simulink model "control"  (R2022b)
settings: Solver=VariableStepAuto  StartTime=0.0  StopTime=4  RelTol=1e-3
undefined symbols (not defined in the file or in its folder): DiscIntNeverNeededParam
libraries: matrix_library x2
settings Model: Creator=giuseppeloianno  LastModifiedBy=reube
settings DataIOCC: ReturnWorkspaceOutputs=off

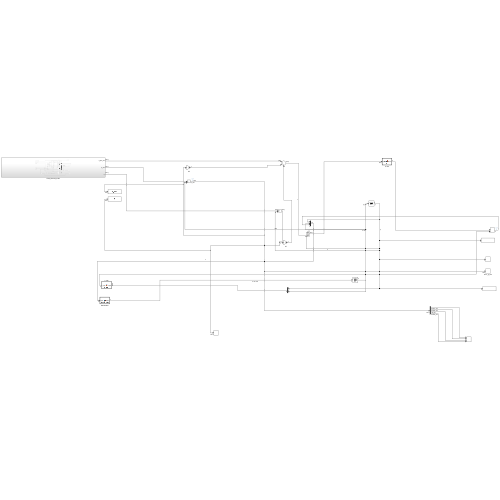
[thumbnail: Simulink's stored preview of the top-level diagram]
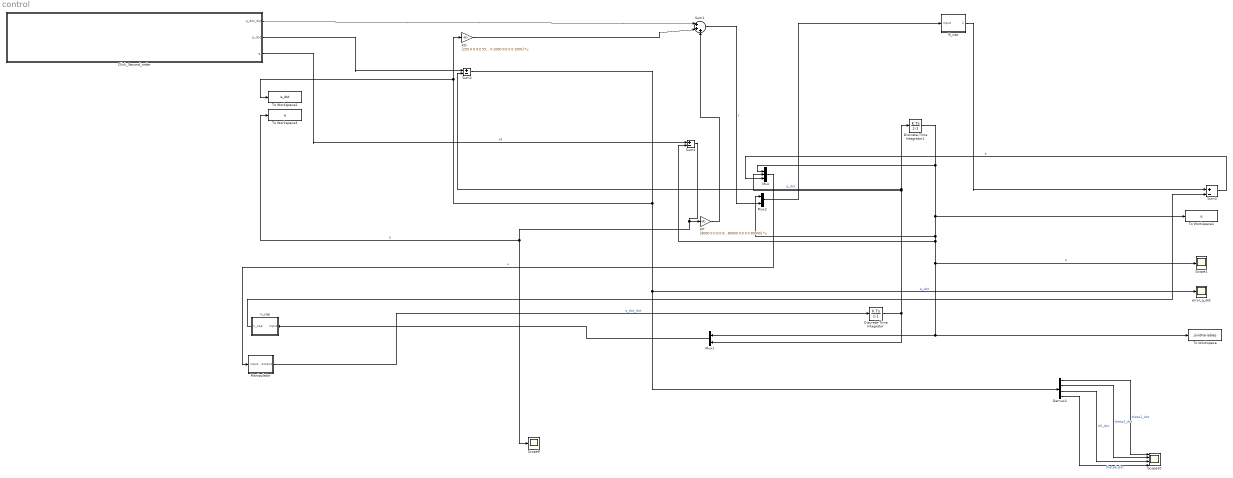
== system control ==
  B_cap : MATLAB Function  TreatAsAtomicUnit=on
  Click_Second_order : Subsystem
  Demux2 : Demux
  Discrete-Time Integrator : DiscreteIntegrator  InitialCondition=[0;0;0;0]  SampleTime=0.001  ICPrevOutput=DiscIntNeverNeededParam  ICPrevScaledInput=DiscIntNeverNeededParam
  Discrete-Time Integrator1 : DiscreteIntegrator  InitialCondition=[-0.9273;-1.2870;0.700;2.2143]  SampleTime=0.001  ICPrevOutput=DiscIntNeverNeededParam  ICPrevScaledInput=DiscIntNeverNeededParam
  KD : Gain  Gain=[250 0 0 0;0 550 0 0;0 0 1000 0;0 0 0 1000]  Multiplication=Matrix(K*u) (u vector)
  KP : Gain  Gain=[8000 0 0 0;0 8000 0 0;0 0 80000 0;0 0 0 80000]  Multiplication=Matrix(K*u) (u vector)
  Manipulator : MATLAB Function  TreatAsAtomicUnit=on
  Mux : Mux  Inputs=3
  Mux1 : Mux  Inputs=2
  Mux2 : Mux  Inputs=2
  Scope1 : Scope
  Scope10 : Scope  NumInputPorts=4
  Scope9 : Scope
  Sum1 : Sum  Inputs=|+++
  Sum2 : Sum  Inputs=|+-
  Sum3 : Sum  Inputs=|+-
  Sum4 : Sum  Inputs=|+-
  To Workspace : ToWorkspace  VariableName=jointVariables  SampleTime=-1
  To Workspace1 : ToWorkspace  VariableName=q  SampleTime=-1
  To Workspace2 : ToWorkspace  VariableName=e_dot  SampleTime=-1
  To Workspace3 : ToWorkspace  VariableName=e  SampleTime=-1
  error_q_dot : Scope
  n_cap : MATLAB Function  TreatAsAtomicUnit=on
  wires:
  Mux/1 -> Manipulator/1(input)  "u"
  Demux2/1 -> Scope10/1  "theta1_dot"
  n_cap/1(n_cap) -> Sum3/2
  Sum1/1 -> Mux2/2  "y"
  B_cap/1(Bmatrixtrue) -> Sum3/1
  Demux2/2 -> Scope10/2  "theta2_dot"
  Sum2/1 -> Demux2/1, error_q_dot/1, To Workspace2/1, KD/1  "e_dot"
  Discrete-Time Integrator1/1 -> Mux1/1, To Workspace/1, Scope1/1, Sum4/2, Mux2/1, To Workspace1/1, Mux/1  "q"
  Mux1/1 -> n_cap/1(input)
  Demux2/3 -> Scope10/3  "d3_dot"
  Manipulator/1(output) -> Discrete-Time Integrator/1  "q_dot_dot"
  Discrete-Time Integrator/1 -> Sum2/2, Discrete-Time Integrator1/1, Mux/2, Mux1/2  "q_dot"
  KD/1 -> Sum1/2
  Click_Second_order/3(q) -> Sum4/1  "xd"
  Sum3/1 -> Mux/3  "e"
  Click_Second_order/2(q_dot) -> Sum2/1
  Sum4/1 -> To Workspace3/1, Scope9/1, KP/1  "e"
  Mux2/1 -> B_cap/1(input)
  Demux2/4 -> Scope10/4  "theta4_dot"
  Click_Second_order/1(q_dot_dot) -> Sum1/1
  KP/1 -> Sum1/3

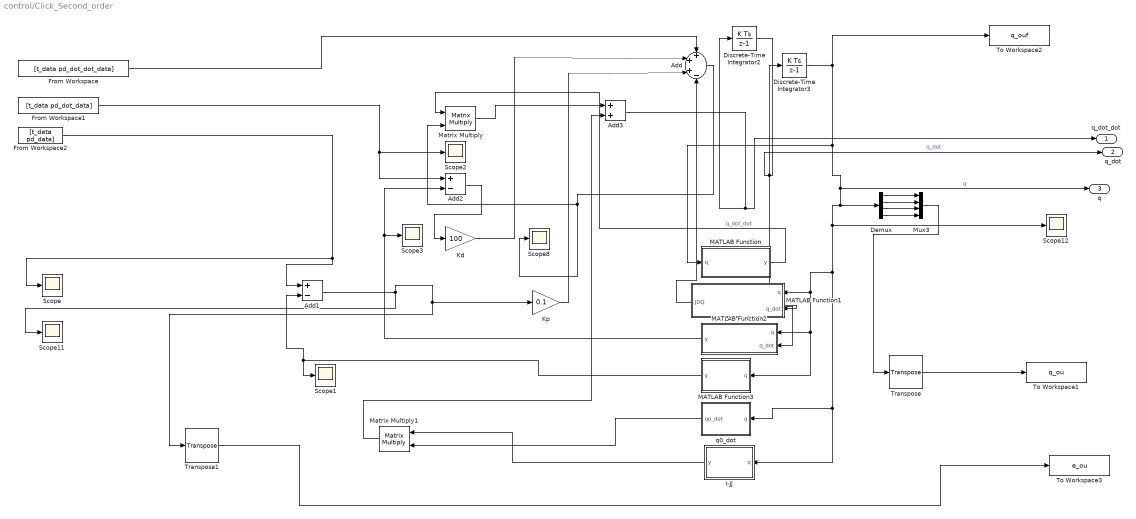
== system control/Click_Second_order ==
  Add : Sum  Inputs=+++-
  Add1 : Sum  Inputs=+-
  Add2 : Sum  Inputs=+-
  Add3 : Sum
  Demux : Demux
  Discrete-Time Integrator2 : DiscreteIntegrator  InitialCondition=[-0.927293431584587;-1.287005790420619;0.700000000000000;2.214299222005206]  SampleTime=0.001  LimitOutput=on  UpperSaturationLimit=[pi/2 pi/4 1 2*pi]'  LowerSaturationLimit="[-pi/2 -pi/2 0.25  -2*pi]'"  ICPrevOutput=DiscIntNeverNeededParam  ICPrevScaledInput=DiscIntNeverNeededParam
  Discrete-Time Integrator3 : DiscreteIntegrator  InitialCondition=[-0.9273;-1.2870;0.700;2.2143]  SampleTime=0.001  LimitOutput=on  UpperSaturationLimit=[pi/2 pi/4 1 2*pi]'  LowerSaturationLimit="[-pi/2 -pi/2 0.25  -2*pi]'"  ICPrevOutput=DiscIntNeverNeededParam  ICPrevScaledInput=DiscIntNeverNeededParam
  From Workspace : FromWorkspace  VariableName=[t_data pd_dot_dot_data]  SampleTime=0.001
  From Workspace1 : FromWorkspace  VariableName=[t_data pd_dot_data]  SampleTime=0.001
  From Workspace2 : FromWorkspace  VariableName=[t_data pd_data]  SampleTime=0.001
  I-JJ : MATLAB Function  TreatAsAtomicUnit=on
  Kd : Gain  Gain=100
  Kp : Gain  Gain=0.1
  MATLAB Function : MATLAB Function  TreatAsAtomicUnit=on
  MATLAB Function1 : MATLAB Function  TreatAsAtomicUnit=on
  MATLAB Function2 : MATLAB Function  TreatAsAtomicUnit=on
  MATLAB Function3 : MATLAB Function  TreatAsAtomicUnit=on
  Matrix Multiply : Product  Multiplication=Matrix(*)
  Matrix Multiply1 : Product  Multiplication=Matrix(*)
  Mux3 : Mux
  Scope{,1..3,8,11..12} (7 alike) : Scope
  To Workspace1 : ToWorkspace  VariableName=q_ou  SampleTime=-1
      settings: Save2DSignal=2-D array (concatenate along first dimension)
  To Workspace2 : ToWorkspace  VariableName=q_ouf  SampleTime=-1
  To Workspace3 : ToWorkspace  VariableName=e_ou  SampleTime=-1
      settings: Save2DSignal=2-D array (concatenate along first dimension)
  Transpose : matrix_library/Transpose
  Transpose1 : matrix_library/Transpose
  q0_dot : MATLAB Function  TreatAsAtomicUnit=on
  q_dot_dot : Outport
  q_dot : Outport  Port=2
  q : Outport  Port=3
  wires:
  Demux/1 -> Mux3/1
  From Workspace/1 -> Add/1
  Demux/2 -> Mux3/2
  Matrix Multiply1/1 -> Add3/2
  Discrete-Time Integrator2/1 -> q_dot/1, MATLAB Function2/2(q_dot), MATLAB Function1/2(q_dot), Discrete-Time Integrator3/1  "q_dot"
  I-JJ/1(y) -> Matrix Multiply1/1
  MATLAB Function1/1(JDQ) -> Add/4
  Add2/1 -> Kd/1
  Kd/1 -> Add/2
  Demux/3 -> Mux3/3
  Matrix Multiply/1 -> Add3/1
  Discrete-Time Integrator3/1 -> q/1, Demux/1, I-JJ/1(q), q0_dot/1(q), MATLAB Function3/1(q), MATLAB Function2/1(q), MATLAB Function1/1(q), Scope12/1, MATLAB Function/1(q), To Workspace2/1  "q"
  Add1/1 -> Transpose1/1, Kp/1, Scope11/1
  MATLAB Function/1(y) -> Matrix Multiply/1  "q_dot_dot"
  MATLAB Function2/1(y) -> Add2/2, Scope3/1
  From Workspace1/1 -> Add2/1, Scope2/1
  From Workspace2/1 -> Add1/1, Scope/1
  Add/1 -> Scope8/1, Matrix Multiply/2
  Kp/1 -> Add/3
  Add3/1 -> Discrete-Time Integrator2/1, q_dot_dot/1
  MATLAB Function3/1(y) -> Add1/2, Scope1/1
  Mux3/1 -> Transpose/1
  Transpose1/1 -> To Workspace3/1
  Transpose/1 -> To Workspace1/1
  Demux/4 -> Mux3/4
  q0_dot/1(qo_dot) -> Matrix Multiply1/2

== matlab function control/Click_Second_order/MATLAB Function ==
  data: q input; y output
function y =pinvj(q)

avariable1 = 0.5;
avariable2 = 0.5;
theta1 = q(1);
theta2 = q(2);
d3 = q(3);
bsum = theta1+theta2;
c1 = cos(theta1);
s1 = sin(theta1);
c12 = cos(bsum);
s12 = sin(bsum);

J = [-avariable2*s12-avariable1*s1 -avariable2*s12 0 0; 
    avariable2*c12+avariable1*c1 avariable2*c12 0 0;  
    0 0 1 0];
x= pinv(J);
y=x;
end

== matlab function control/Click_Second_order/MATLAB Function2 ==
  data: q input; q_dot input; y output
function y = jacobian(q, q_dot)
a1 = 0.5;
a2 = 0.5;
t1 = q(1);
t2 = q(2);
d3 = q(3);
b = t1+t2;
c1 = cos(t1);
s1 = sin(t1);
c12 = cos(b);
s12 = sin(b);


J = [-a2*s12-a1*s1 -a2*s12 0 0; 
    a2*c12+a1*c1 a2*c12 0 0;  
    0 0 -1.5+d3 0];
y = J*q_dot;

end

== matlab function control/Click_Second_order/MATLAB Function3 ==
  data: q input; y output
function y = direct_kin(q)
aSIDE1=0.5;
aSIDE2=0.5;
tETA1=q(1);
tETA2=q(2);
b=tETA1+tETA2;
d3side=q(3);
ct1= cos(tETA1);
st1 = sin(tETA1);
ct12 = cos(b);
st12 = sin(b);
y=[aSIDE2*ct12+aSIDE1*ct1;
   aSIDE1*st12 + aSIDE1*st1;
   -1.5+d3side];
end

== matlab function control/Click_Second_order/I-JJ ==
  data: q input; y output
function y = ijj(q)


aside1 = 0.5;
aside2 = 0.5;
theta1 = q(1);
theta2 = q(2);
d3 = q(3);
bsum = theta1+theta2;
c1 = cos(theta1);
s1 = sin(theta1);
c12 = cos(bsum);
s12 = sin(bsum);
k = 10;

Jacobian = [-aside2*s12-aside1*s1 -aside2*s12 0 0; 
    aside2*c12+aside1*c1 aside2*c12 0 0;  
    0 0 1 0];
x= pinv(Jacobian);


c = [1 0 0 0; 0 1 0 0; 0 0 1 0; 0 0 0 1] - (x * Jacobian);

%p=[0.4;-0.7;0.5;1];


%q_dotmatrix=[-(2*(sin(bsum)/2 + sin(q(1))/2)*(cos(bsum)/2 + cos(q(1))/2 - p(1,:)) - 2*(cos(bsum)/2 + cos(q(1))/2)*(sin(bsum)/2 + sin(q(1))/2 + p(2,:)))/(2*((cos(bsum)/2 + cos(q(1))/2 - p(1,:))^2 + (sin(bsum)/2 + sin(q(1))/2 + p(2,:))^2 + (q(3) - p(3,:))^2)^(1/2)),  -(sin(bsum)*(cos(bsum)/2 + cos(q(1))/2 - p(1,:)) - cos(bsum)*(sin(bsum)/2 + sin(q(1))/2 + p(2,:)))/(2*((cos(bsum)/2 + cos(q(1))/2 - p(1,:))^2 + (sin(bsum)/2 + sin(q(1))/2 + p(2,:))^2 + (q(3) - p(3,:))^2)^(1/2)),  (2*q(3) - 1)/(2*((cos(bsum)/2 + cos(q(1))/2 - p(1,:))^2 + (sin(bsum)/2 + sin(q(1))/2 + p(2,:))^2 + (q(3) - p(3,:))^2)^(1/2)), 0];


%g =k* q_dotmatrix.';

y = c ;
end

== matlab function control/Click_Second_order/q0_dot ==
  data: q input; qo_dot output
function qo_dot = qodot(q)


aside1 = 0.5;
aside2 = 0.5;
theta1 = q(1);
theta2 = q(2);
t3 = q(3);
b = theta1+theta2;
cside1 = cos(theta1);
sside1 = sin(theta1);
cside12 = cos(b);
sside12 = sin(b);
k = 10;

J = [-aside2*sside12-aside1*sside1 -aside2*sside12 0 0; 
    aside2*cside12+aside1*cside1 aside2*cside12 0 0;  
    1 1 0 1];
x= pinv(J);


c = [1 0 0 0; 0 1 0 0; 0 0 1 0; 0 0 0 1] - (x * J);

p=[0.4;-0.7;0.5;1];
p1= p(1);
p2=p(2);
p3=p(3);

qo_dot=k * [(-q(1)/(4*(pi)^2));(-4/(9*(pi)^2))*(q(2)+(pi*8));(0.625-q(3))/2.25;-q(4)/(16*(pi)^2)];

end

== matlab function control/B_cap ==
  data: input input; Bmatrixtrue output
function  Bmatrixtrue = B(input)
    t2=input(2,:);
    yinput1=input(5,:);
    yinput2=input(6,:);
    yinput3=input(7,:);    
    yinput4=input(8,:);
    massl1 = 25;
    massl2 = 25;
    massl3 = 10;
    massl4 = 0;
    Ilink1 = 5;
    Ilink2 = 5;
    Ilink4 = 1;
    Imass1 = 0.0001;
    Imass2 = 0.0001;
    Imass3 = 0.01;
    Imass4 = 0.005;
    l1 = 0.25;
    l2 = 0.25;
    kinetic1 = 1;
    kinetic2 = 1;
    kinetic3 = 50;
    kinetic4 = 20;
    g = 9.8;
    b11=l1^2*massl1+(0.25+l2^2+l2*cos(t2))*massl2+(0.5+0.5*cos(t2))*(massl3+massl4)+Ilink1+Ilink2+Ilink4+Imass1*kinetic1^2+Imass2+Imass3+Imass4;
    b12=(0.5*l2*cos(t2)+l2^2)*massl2+(0.25+0.25*cos(t2))*(massl3+massl4)+Ilink2+Ilink4+Imass2*kinetic2++Imass3+Imass4;
    b13=-kinetic3*Imass3;
    b14=kinetic4*Imass4+Ilink4;
    b21=b12;
    b22=l2^2*massl2+0.25*(massl4+massl3)+Ilink2+Ilink4+Imass2*kinetic2^2+Imass4+Imass3;
    b23=-kinetic3*Imass3;
    b24=kinetic4*Imass4+Ilink4;
    b31=b13;
    b32=b23;
    b33=Imass3*kinetic3^2+massl3+massl4;
    b34=0;
    b41=b14;
    b42=b24;
    b43=b34;
    b44=Imass4*kinetic4^2+Ilink4;
    Bmatrixt=[b11 b12 b13 b14; b21 b22 b23 b24; b31 b32 b33 b34; b41 b42 b43 b44];
    Bmatrixtrue=Bmatrixt*transpose([yinput1 yinput2 yinput3 yinput4]);
end

== matlab function control/Manipulator ==
  data: input input; output output
function output = Manipulator(input)
% Part 2 manipulatort2d
   t1 = input(1,:);
    t2 = input(2,:);
    d3 = input(3,:);
    t4 = input(4,:);
    t1d = input(5,:);
    t2d = input(6,:);
    d3d = input(7,:);
    t4d = input(8,:);
    ip1 = input(9,:);
    ip2 = input(10,:);
    ip3 = input(11,:);
    ip4 = input(12,:);
    massl1 = 25;
    massl2 = 25;
    massl3 = 10;
    massl4 = 5;
    Ilink1 = 5;
    Ilink2= 5;
    Ilink4= 1;
    IMass1 = 0.0001;
    IMass2 = 0.0001;
    IMass3 = 0.01;
    IMass4 = 0.005;
    link1 = 0.25;
    link2 = 0.25;
    kr1 = 1;
    kr2 = 1;
    kr3 = 50;
    kr4 = 20;
    gravity = 9.8;
    Forcev11 = 0.0001;
    Forcev22 = 0.0001;
    Forcev33 = 0.01;
    Forcev44 = 0.005;
    
    b11=link1^2*massl1+(0.25+link2^2+link2*cos(t2))*massl2+(0.5+0.5*cos(t2))*(massl3+massl4)+Ilink1+Ilink2+Ilink4+IMass1*kr1^2+IMass2+IMass3+IMass4;
    b12=(0.5*link2*cos(t2)+link2^2)*massl2+(0.25+0.25*cos(t2))*(massl3+massl4)+Ilink2+Ilink4+IMass2*kr2++IMass3+IMass4;
    b13=-kr3*IMass3;
    b14=kr4*IMass4+Ilink4;
    b21=b12;
    b22=link2^2*massl2+0.25*(massl4+massl3)+Ilink2+Ilink4+IMass2*kr2^2+IMass4+IMass3;
    b23=-kr3*IMass3;
    b24=kr4*IMass4+Ilink4;
    b31=b13;
    b32=b23;
    b33=IMass3*kr3^2+massl3+massl4;
    b34=0;
    b41=b14;
    b42=b24;
    b43=b34;
    b44=IMass4*kr4^2+Ilink4;
    Bmatrix=[b11 b12 b13 b14; b21 b22 b23 b24; b31 b32 b33 b34; b41 b42 b43 b44];
    Cmatrix=[(-link2*massl2*sin(t2)-0.5*(massl4+massl3)*sin(t2))/2*t2d (-link2*massl2*sin(t2)-0.5*(massl4+massl3)*sin(t2))/2*(t1d+t2d) 0 0;
    -(-link2*massl2*sin(t2)-0.5*(massl4+massl3)*sin(t2))/2*t1d 0 0 0; 0 0 0 0; 0 0 0 0];
    Gmatrix = [0; 0; -(massl3+massl4)*gravity; 0];
    F = diag([kr1^2*Forcev11 kr2^2*Forcev22 kr3^2*Forcev33 kr4^2*Forcev44]);
    
    tou = [ip1 ip2 ip3 ip4]';
    tou_1 = Cmatrix*[t1d t2d d3d t4d]'+F*[t1d t2d d3d t4d]'+Gmatrix;
    
    q_dot_dot = inv(Bmatrix)*(tou-tou_1);
    
    output = q_dot_dot;
   
end

== matlab function control/n_cap ==
  data: input input; n_cap output
function n_cap  = n_cap(input)
    t2=input(2,:);
    t1d=input(5,:);
    t2d=input(6,:);
    d3d=input(7,:);
    t4d=input(8,:);
    massl2 = 25;
    massl3 = 10;
    massl4 = 0;
    length2 = 0.25;
    kinetic1 = 1;
    kinetic2 = 1;
    kinetic3 = 50;
    kinetic4 = 20;
    g = 9.8;
    forcev1 = 0.0001;
    forcev2 = 0.0001;
    forcev3 = 0.01;
    forcev4 = 0.005;
    Cc=[(-length2*massl2*sin(t2)-0.5*(massl4+massl3)*sin(t2))/2*t2d (-length2*massl2*sin(t2)-0.5*(massl4+massl3)*sin(t2))/2*(t1d+ t2d) 0 0;
    -(-length2*massl2*sin(t2)-0.5*(massl4+massl3)*sin(t2))/2*t1d 0 0 0; 0 0 0 0; 0 0 0 0];
    Gvector = [0; 0; -(massl3+massl4)*g; 0];
    Fvector = diag([kinetic1^2*forcev1 kinetic2^2*forcev2 kinetic3^2*forcev3 kinetic4^2*forcev4]);
    n_cap = Cc*[t1d t2d d3d t4d]'+Fvector*[t1d t2d d3d t4d]'+Gvector;
end

== matlab function control/Click_Second_order/MATLAB Function1 ==
  data: q input; q_dot input; JDQ output
function JDQ = jacobian_ddot(q,q_dot)
theta1 = q(1);
theta2 = q(2);


theta1_dot = q_dot(1);
theta2_dot = q_dot(2);


wa1 = (cos(theta1)*theta1_dot)/2;
xa1 = (sin(theta1)*theta1_dot)/2;
ya1 = (sin(theta1 + theta2)*(theta1_dot + theta2_dot))/2;
za1 = (cos(theta1 + theta2)*(theta1_dot + theta2_dot))/2;

Jd = [-wa1-za1 -za1 0 0;
    -xa1-ya1 -ya1 0 0;
    0 0 0 0
];
JDQ = Jd*q_dot;

end
